simulink model "simulation_homework2"  (R2020b)
settings: Solver=VariableStepAuto  StartTime=0.0  StopTime=10  RelTol=1e-3
values from neighbouring files (symbols this model uses):
  F1 = Ys1 * inv(Xs)    [homework2.m]    (also in inverted_pendulum_fuzzy.m)
  F2 = Ys2 * inv(Xs)    [homework2.m]    (also in inverted_pendulum_fuzzy.m)
  g = 9.8    [homework2.m]    (also in inverted_pendulum_fuzzy.m)
  I = 1    [homework2.m]    (also in inverted_pendulum_fuzzy.m)
  Initial_angle1 = 90    [homework2.m]    (also in inverted_pendulum_fuzzy.m)
  Initial_angle2 = 60    [homework2.m]    (also in inverted_pendulum_fuzzy.m)
  input = [180 160 0 0]'    [homework2.m]    (also in inverted_pendulum_fuzzy.m = [0 0 0 0]')
  J = 1    [homework2.m]    (also in inverted_pendulum_fuzzy.m)
  k = 100    [homework2.m]    (also in inverted_pendulum_fuzzy.m)
  L = 1    [homework2.m]    (also in inverted_pendulum_fuzzy.m)
  m = 1    [homework2.m]    (also in inverted_pendulum_fuzzy.m)
settings Model: Creator=seo27  LastModifiedBy=seo27

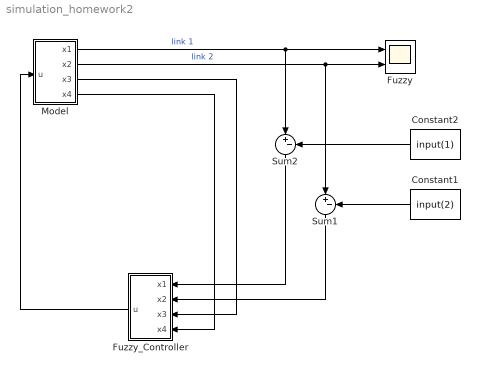
== system simulation_homework2 ==
  Constant1 : Constant  Value=input(2)
  Constant2 : Constant  Value=input(1)
  Fuzzy : Scope  NumInputPorts=2
  Fuzzy_Controller : Subsystem
  Model : Subsystem
  Sum1 : Sum  Inputs=|+-
  Sum2 : Sum  Inputs=|+-
  wires:
  Model/2(x2) -> Fuzzy/2, Sum1/1  "link 2"
  Model/1(x1) -> Sum2/1, Fuzzy/1  "link 1"
  Model/4(x4) -> Fuzzy_Controller/4(x4)
  Model/3(x3) -> Fuzzy_Controller/3(x3)
  Fuzzy_Controller/1(u) -> Model/1(u)
  Constant1/1 -> Sum1/2
  Sum1/1 -> Fuzzy_Controller/2(x2)
  Sum2/1 -> Fuzzy_Controller/1(x1)
  Constant2/1 -> Sum2/2

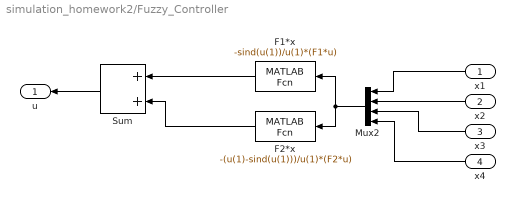
== system simulation_homework2/Fuzzy_Controller ==
  x1 : Inport
  x2 : Inport  Port=2
  x3 : Inport  Port=3
  x4 : Inport  Port=4
  F1*x : MATLABFcn  MATLABFcn=-sind(u(1))/u(1)*(F1*u)
  F2*x : MATLABFcn  MATLABFcn=-(u(1)-sind(u(1)))/u(1)*(F2*u)
  Mux2 : Mux
  Sum : Sum
  u : Outport
  wires:
  Sum/1 -> u/1
  x1/1 -> Mux2/1
  x2/1 -> Mux2/2
  Mux2/1 -> F2*x/1, F1*x/1
  F1*x/1 -> Sum/1
  F2*x/1 -> Sum/2
  x3/1 -> Mux2/3
  x4/1 -> Mux2/4

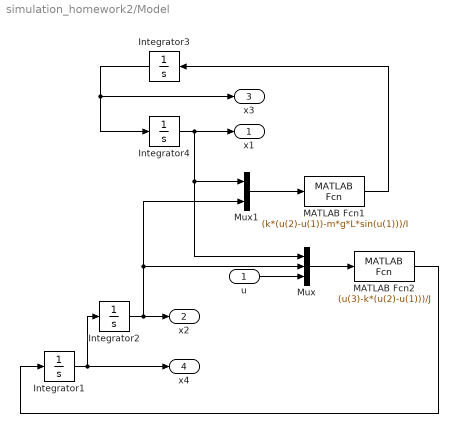
== system simulation_homework2/Model ==
  u : Inport
  Integrator1 : Integrator
  Integrator2 : Integrator  InitialCondition=Initial_angle2
  Integrator3 : Integrator
  Integrator4 : Integrator  InitialCondition=Initial_angle1
  MATLAB Fcn1 : MATLABFcn  MATLABFcn=(k*(u(2)-u(1))-m*g*L*sin(u(1)))/I
  MATLAB Fcn2 : MATLABFcn  MATLABFcn=(u(3)-k*(u(2)-u(1)))/J
  Mux : Mux  Inputs=3
  Mux1 : Mux  Inputs=2
  x1 : Outport
  x2 : Outport  Port=2
  x3 : Outport  Port=3
  x4 : Outport  Port=4
  wires:
  Integrator1/1 -> Integrator2/1, x4/1
  Mux1/1 -> MATLAB Fcn1/1
  MATLAB Fcn1/1 -> Integrator3/1
  Integrator4/1 -> x1/1, Mux1/1, Mux/1
  Mux/1 -> MATLAB Fcn2/1
  MATLAB Fcn2/1 -> Integrator1/1
  Integrator3/1 -> Integrator4/1, x3/1
  u/1 -> Mux/3
  Integrator2/1 -> x2/1, Mux1/2, Mux/2
